simulink model "LAB2_2_Body_problem"  (R2022b)
settings: Solver=FixedStepAuto  StartTime=t0  StopTime=tf  FixedStep=0.1  RelTol=1e-3
values from neighbouring files (symbols this model uses):
  mu_sun = 1.327e11    (= 132700000000)    [LAB_02.m]
  r0 = [2.029e8; -1.475e5; -1.1395e7]    [LAB_02.m]
  v0 = [3.021; 24.139; 10.964]    [LAB_02.m]
settings Model: Creator=ludov  LastModifiedBy=ludov

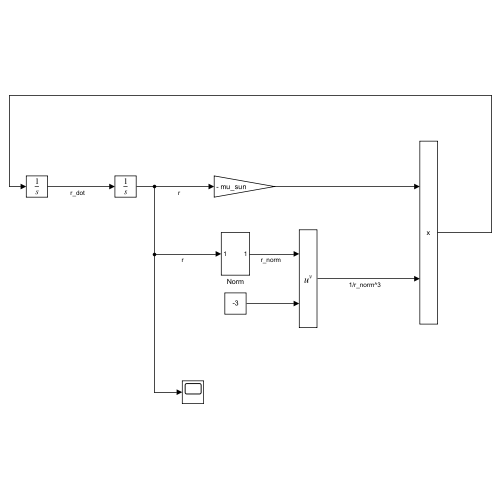
[thumbnail: Simulink's stored preview of the top-level diagram]
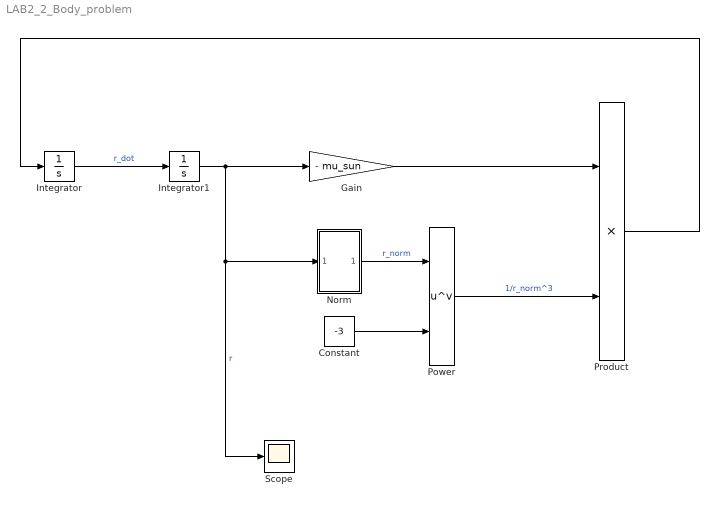
== system LAB2_2_Body_problem ==
  Constant : Constant  Value=-3
  Gain : Gain  Gain=- mu_sun
  Integrator : Integrator  InitialCondition=v0
  Integrator1 : Integrator  InitialCondition=r0
  Norm : Subsystem
  Power : Math  Operator=pow
  Product : Product
  Scope : Scope
  wires:
  Integrator/1 -> Integrator1/1  "r_dot"
  Integrator1/1 -> Scope/1, Norm/1(In1), Gain/1  "r"
  Norm/1(Out1) -> Power/1  "r_norm"
  Constant/1 -> Power/2
  Power/1 -> Product/2  "1/r_norm^3"
  Gain/1 -> Product/1
  Product/1 -> Integrator/1

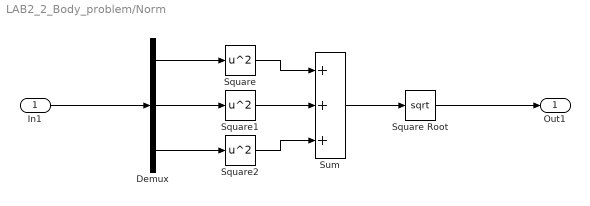
== system LAB2_2_Body_problem/Norm ==
  In1 : Inport
  Demux : Demux  Outputs=3
  Square : Math  Operator=square
  Square Root : Sqrt
  Square1 : Math  Operator=square
  Square2 : Math  Operator=square
  Sum : Sum  Inputs=+++
  Out1 : Outport
  wires:
  Demux/3 -> Square2/1
  Sum/1 -> Square Root/1
  Demux/1 -> Square/1
  Square1/1 -> Sum/2
  Demux/2 -> Square1/1
  In1/1 -> Demux/1
  Square2/1 -> Sum/3
  Square/1 -> Sum/1
  Square Root/1 -> Out1/1
